simulink model "LAB1_P4"  (R2024a)
settings: Solver=VariableStepAuto  StartTime=0.0  StopTime=100  RelTol=1e-3
settings Model: Creator=Sarst  LastModifiedBy=Sarst

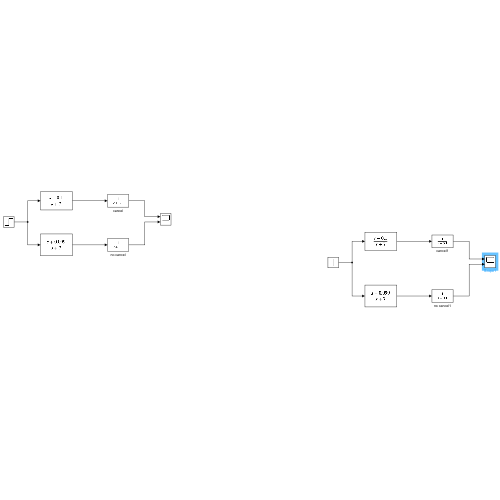
[thumbnail: Simulink's stored preview of the top-level diagram]
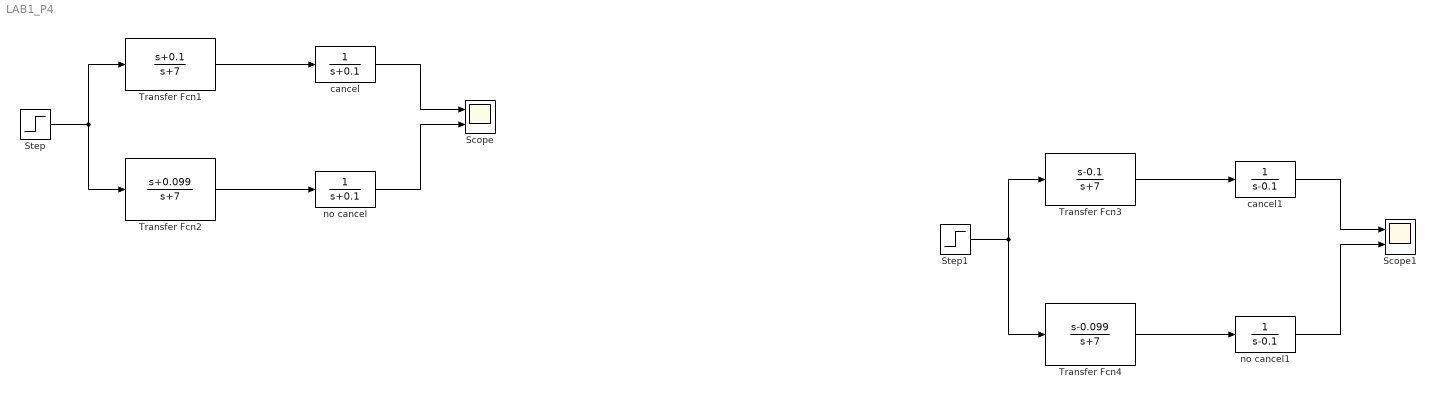
== system LAB1_P4 ==
  Scope : Scope  NumInputPorts=2
  Scope1 : Scope  NumInputPorts=2
  Step : Step  Time=0  SampleTime=0
  Step1 : Step  Time=0  SampleTime=0
  Transfer Fcn1 : TransferFcn  Numerator=[1 0.1]  Denominator=[1 7]
  Transfer Fcn2 : TransferFcn  Numerator=[1 0.099]  Denominator=[1 7]
  Transfer Fcn3 : TransferFcn  Numerator=[1 -0.1]  Denominator=[1 7]
  Transfer Fcn4 : TransferFcn  Numerator=[1 -0.099]  Denominator=[1 7]
  cancel : TransferFcn  Denominator=[1 0.1]
  cancel1 : TransferFcn  Denominator=[1 -0.1]
  no cancel : TransferFcn  Denominator=[1 0.1]
  no cancel1 : TransferFcn  Denominator=[1 -0.1]
  wires:
  Transfer Fcn1/1 -> cancel/1
  Step/1 -> Transfer Fcn1/1, Transfer Fcn2/1
  Transfer Fcn2/1 -> no cancel/1
  cancel/1 -> Scope/1
  no cancel/1 -> Scope/2
  cancel1/1 -> Scope1/1
  Transfer Fcn3/1 -> cancel1/1
  Step1/1 -> Transfer Fcn4/1, Transfer Fcn3/1
  Transfer Fcn4/1 -> no cancel1/1
  no cancel1/1 -> Scope1/2
